simulink model "OFDM_Tx_HW"  (R2020a)
settings: Solver=FixedStepDiscrete  StartTime=0.0  StopTime=inf  RelTol=1e-3
InitFcn:
  | % Set parameters
  | fs = 20e6;
  | fclk = 240e6;
  | ssr = 2;
  | fdc = fclk*ssr*8;
  | 
  | % Load libraries
  | addpath('./lib');
  | 
  | % Create filters
  | run ./filter_design_20mhz;
  | 
  | % Load all required variables
  | load('variables/read_addr_data');
  | load('variables/read_addr_cp');
  | load('variables/read_addr_pream');
  | load('variables/read_addr_rx');
  | load('variables/pilot');
  | load('variables/sc_index');
  | load('variables/LTSfreq');
  | load('variables/STSfreq');
  | load('variables/LTSread');
  | load('variables/STSread');
  | 
  | run ./scripts/rfgen;
values from neighbouring files (symbols this model uses):
  decimation_unique = dsp.SampleRateConverter('InputSampleRate', fdc/64,     'OutputSampleRate', fs,     'Bandwidth', fs*0.9,     'OutputRateTolerance', 0,     'StopbandAttenuation', 100)    [filter_design_20mhz.m]
  interpolation_single = dsp.SampleRateConverter('InputSampleRate', fs,     'OutputSampleRate', fclk,     'Bandwidth', fs*0.9,     'OutputRateTolerance', 0,     'StopbandAttenuation', 100)    [filter_design_20mhz.m]
  interpolation_ssr = dsp.SampleRateConverter('InputSampleRate', fclk,     'OutputSampleRate', fclk*ssr,     'Bandwidth', fs*0.9,     'OutputRateTolerance', 0,     'StopbandAttenuation', 100)    [filter_design_20mhz.m]
undefined symbols (not defined in the file or in its folder): designMultirateFIR, LTSfreq, LTSread, pilot, read_addr_cp, read_addr_data, read_addr_pream, read_addr_rx, sc_index, STSfreq, STSread
libraries: hdlsllib x87, simulink x55, xbsIndex_r4 x48, dspmlti4 x23, xrbsSSR_Library x8, dspsigops x6, dspswit3 x4, dsphdlmathfun x3, dspsigattribs x2, dsphdlxfrm x2, dsphdlsigops x1, lib_rfsignalgenerator x1
(part 6 of 6)

== system OFDM_Tx_HW/OFDMTx/CPAdd/LTFExtend/LTFValidGen ==
  In1 : Inport
  AND : Logic  IconShape=distinctive  AllPortsSameDT=off  OutDataTypeStr=boolean
  AND1 : Logic  IconShape=distinctive  AllPortsSameDT=off  OutDataTypeStr=boolean
  Compare To Constant : simulink/Logic and Bit Operations/Compare To Constant  relop=>=  const=160  OutDataTypeStr=boolean
  Compare To Constant1 : simulink/Logic and Bit Operations/Compare To Constant  relop=<=  const=319  OutDataTypeStr=boolean
  HDL Counter : hdlsllib/Sources/HDL Counter  CountType=Count limited  CountInit=0  CountStep=1  CountMax=319  CountFromType=Initial value  CountFrom=0  CountResetPort=on  CountLoadPort=off  CountEnbPort=on  CountDirPort=off  CountDataType=Unsigned  CountWordLen=9  CountFracLen=0  CountSampTime=1
  NOT : Logic  Operator=NOT  IconShape=distinctive  AllPortsSameDT=off  OutDataTypeStr=boolean
  Out1 : Outport  VectorParamsAs1DForOutWhenUnconnected=off
  wires:
  Compare To Constant/1 -> AND/1
  In1/1 -> NOT/1, AND1/2, HDL Counter/2
  HDL Counter/1 -> Compare To Constant1/1, Compare To Constant/1
  Compare To Constant1/1 -> AND/2
  AND1/1 -> Out1/1
  AND/1 -> AND1/1
  NOT/1 -> HDL Counter/1

== system OFDM_Tx_HW/OFDMTx/CPAdd/LTFExtend/READ_CTRL ==
  In1 : Inport
  In2 : Inport  Port=2
  Constant : Constant  Value=0  OutDataTypeStr=fixdt(0,8,0)  SampleTime=1/fs
  Switch : Switch  Criteria=u2 ~= 0
  Out1 : Outport  VectorParamsAs1DForOutWhenUnconnected=off
  wires:
  Switch/1 -> Out1/1
  In1/1 -> Switch/1
  In2/1 -> Switch/2
  Constant/1 -> Switch/3

== system OFDM_Tx_HW/OFDMTx/CPAdd/STFExtend/READ_CTRL ==
  In1 : Inport
  In2 : Inport  Port=2
  Constant : Constant  Value=0  OutDataTypeStr=fixdt(0,8,0)  SampleTime=1/fs
  Switch : Switch  Criteria=u2 ~= 0
  Out1 : Outport  VectorParamsAs1DForOutWhenUnconnected=off
  wires:
  Constant/1 -> Switch/3
  In2/1 -> Switch/2
  In1/1 -> Switch/1
  Switch/1 -> Out1/1

== system OFDM_Tx_HW/OFDMTx/CPAdd/STFExtend/STFValidGen ==
  In1 : Inport
  AND : Logic  IconShape=distinctive  AllPortsSameDT=off  OutDataTypeStr=boolean
  AND1 : Logic  IconShape=distinctive  AllPortsSameDT=off  OutDataTypeStr=boolean
  Compare To Constant : simulink/Logic and Bit Operations/Compare To Constant  relop=>=  const=0  OutDataTypeStr=boolean
  Compare To Constant1 : simulink/Logic and Bit Operations/Compare To Constant  relop=<=  const=159  OutDataTypeStr=boolean
  HDL Counter : hdlsllib/Sources/HDL Counter  CountType=Count limited  CountInit=0  CountStep=1  CountMax=319  CountFromType=Initial value  CountFrom=0  CountResetPort=on  CountLoadPort=off  CountEnbPort=on  CountDirPort=off  CountDataType=Unsigned  CountWordLen=9  CountFracLen=0  CountSampTime=1
  NOT : Logic  Operator=NOT  IconShape=distinctive  AllPortsSameDT=off  OutDataTypeStr=boolean
  Out1 : Outport  VectorParamsAs1DForOutWhenUnconnected=off
  wires:
  Compare To Constant/1 -> AND/1
  In1/1 -> NOT/1, AND1/2, HDL Counter/2
  HDL Counter/1 -> Compare To Constant1/1, Compare To Constant/1
  Compare To Constant1/1 -> AND/2
  AND1/1 -> Out1/1
  AND/1 -> AND1/1
  NOT/1 -> HDL Counter/1

== system OFDM_Tx_HW/OFDMTx/ControlSignalGenerator/PreamValidGen/RisingEdge ==
  In1 : Inport
  Delay : Delay  DelayLength=1
  Relational Operator : RelationalOperator  Operator=>  OutDataTypeStr=boolean  RndMeth=Nearest
  Out1 : Outport
  wires:
  Relational Operator/1 -> Out1/1
  Delay/1 -> Relational Operator/2
  In1/1 -> Delay/1, Relational Operator/1

== system OFDM_Tx_HW/OFDMTx/DataGenerator/PilotGen/ToComplex1 ==
  In1 : Inport
  Constant1 : Constant  Value=0  OutDataTypeStr=fixdt(1,16,14)  SampleTime=1/fs
  Real-Imag to Complex : RealImagToComplex
  PilotOut : Outport  VectorParamsAs1DForOutWhenUnconnected=off
  wires:
  Constant1/1 -> Real-Imag to Complex/2
  In1/1 -> Real-Imag to Complex/1
  Real-Imag to Complex/1 -> PilotOut/1

== system OFDM_Tx_HW/OFDMTx/IFFT/IFFTValid/dataIFFTValid ==
  dataValidIn : Inport
  Compare To Constant : simulink/Logic and Bit Operations/Compare To Constant  relop=>=  const=17  OutDataTypeStr=boolean
  Logical Operator : Logic  Operator=NOT  IconShape=distinctive  AllPortsSameDT=off  OutDataTypeStr=boolean
  SAMPLE_COUNTER : hdlsllib/Sources/HDL Counter  CountType=Count limited  CountInit=1  CountStep=1  CountMax=80  CountFromType=Initial value  CountFrom=1  CountResetPort=on  CountLoadPort=off  CountEnbPort=on  CountDirPort=off  CountDataType=Unsigned  CountWordLen=7  CountFracLen=0  CountSampTime=1
  dataIFFTValidOut : Outport  VectorParamsAs1DForOutWhenUnconnected=off
  wires:
  dataValidIn/1 -> SAMPLE_COUNTER/2, Logical Operator/1
  Compare To Constant/1 -> dataIFFTValidOut/1
  Logical Operator/1 -> SAMPLE_COUNTER/1
  SAMPLE_COUNTER/1 -> Compare To Constant/1

== system OFDM_Tx_HW/OFDMTx/IFFT/IFFTValid/preambIFFTValid ==
  preambValid : Inport
  AND{,1..3} (4 alike) : Logic  IconShape=distinctive  AllPortsSameDT=off  OutDataTypeStr=boolean
  Compare To Constant1 : simulink/Logic and Bit Operations/Compare To Constant  relop=>=  const=96  OutDataTypeStr=boolean
  Compare To Constant2 : simulink/Logic and Bit Operations/Compare To Constant  relop=<=  const=159  OutDataTypeStr=boolean
  Compare To Constant3 : simulink/Logic and Bit Operations/Compare To Constant  relop=>=  const=256  OutDataTypeStr=boolean
  Compare To Constant4 : simulink/Logic and Bit Operations/Compare To Constant  relop=<=  const=319  OutDataTypeStr=boolean
  HDL Counter1 : hdlsllib/Sources/HDL Counter  CountType=Count limited  CountInit=0  CountStep=1  CountMax=319  CountFromType=Initial value  CountFrom=0  CountResetPort=on  CountLoadPort=off  CountEnbPort=on  CountDirPort=off  CountDataType=Unsigned  CountWordLen=9  CountFracLen=0  CountSampTime=1
  NOT : Logic  Operator=NOT  IconShape=distinctive  AllPortsSameDT=off  OutDataTypeStr=boolean
  OR : Logic  Operator=OR  IconShape=distinctive  AllPortsSameDT=off  OutDataTypeStr=boolean
  preambIFFTValidOut : Outport  VectorParamsAs1DForOutWhenUnconnected=off
  wires:
  AND/1 -> AND1/1
  AND2/1 -> AND3/1
  HDL Counter1/1 -> Compare To Constant4/1, Compare To Constant3/1, Compare To Constant2/1, Compare To Constant1/1
  OR/1 -> preambIFFTValidOut/1
  preambValid/1 -> HDL Counter1/2, AND3/2, AND1/2, NOT/1
  Compare To Constant1/1 -> AND/1
  Compare To Constant4/1 -> AND2/2
  AND1/1 -> OR/1
  AND3/1 -> OR/2
  Compare To Constant2/1 -> AND/2
  NOT/1 -> HDL Counter1/1
  Compare To Constant3/1 -> AND2/1

== system OFDM_Tx_HW/OFDMTx/SCMapper/DataMapper/READ_CTRL2 ==
  In1 : Inport
  In2 : Inport  Port=2
  Constant : Constant  Value=0  OutDataTypeStr=fixdt(0,8,0)  SampleTime=1/fs
  Switch : Switch  Criteria=u2 ~= 0
  Out1 : Outport  VectorParamsAs1DForOutWhenUnconnected=off
  wires:
  Switch/1 -> Out1/1
  In1/1 -> Switch/1
  In2/1 -> Switch/2
  Constant/1 -> Switch/3

== system OFDM_Tx_HW/OFDMTx/SCMapper/PremableMapper/READ_CTRL ==
  In1 : Inport
  In2 : Inport  Port=2
  Constant : Constant  Value=0  OutDataTypeStr=fixdt(0,8,0)  SampleTime=1/fs
  Switch : Switch  Criteria=u2 ~= 0
  Out1 : Outport  VectorParamsAs1DForOutWhenUnconnected=off
  wires:
  Switch/1 -> Out1/1
  In1/1 -> Switch/1
  In2/1 -> Switch/2
  Constant/1 -> Switch/3

== system OFDM_Tx_HW/decimate/Unique Decimation/Unique Decimation/FIR Decimator Unique ==
  Re Data In : Inport
  Im Data In : Inport  Port=2
  Convert7 : xbsIndex_r4/Convert  gui_display_data_type=Fixed-point  arith_type="Signed  (2's comp)"  n_bits=16  bin_pt=14  float_type=Single  exp_bits=8  fraction_bits=24  quantization="Round  (unbiased: +/- Inf)"  overflow=Saturate  en=off  latency=0  pipeline=off  dbl_ovrd=off  block_type=convert
  Convert8 : xbsIndex_r4/Convert  gui_display_data_type=Fixed-point  arith_type="Signed  (2's comp)"  n_bits=16  bin_pt=14  float_type=Single  exp_bits=8  fraction_bits=24  quantization="Round  (unbiased: +/- Inf)"  overflow=Saturate  en=off  latency=0  pipeline=off  dbl_ovrd=off  block_type=convert
  FIR Stage Unique : xbsIndex_r4/FIR Compiler 7.2   coefficientvector=decimation_unique.getFilters.Stage1.Numerator  coefficient_sets=1  coefficient_reload=off  filter_type=Decimation  rate_change_type=Integer  interpolation_rate=1  decimation_rate=decimation_unique.getFilters.Stage1.DecimationFactor  zero_pack_factor=1  channel_sequence=Basic  number_channels=1  pattern_list='P4-0,P4-1,P4-2,P4-3,P4-4'  number_paths=2  ratespecification=Maximum_Possible  sampleperiod=3  hardwareoversamplingrate=1  coefficient_sign=Signed  quantization=Quantize_Only  coefficient_width=16  bestprecision=on  coefficient_fractional_bits=16  coefficient_structure=Inferred  output_rounding_mode=Full_Precision  output_width=34  filter_architecture=Systolic_Multiply_Accumulate  optimization_goal=Area  optimization_list='None'  data_buffer_type=Automatic  coefficient_buffer_type=Automatic  input_buffer_type=Automatic  output_buffer_type=Automatic  preference_for_other_storage=Automatic  multi_column_support=Automatic  columnconfig='33'  inter_column_pipe_length=4  data_has_tlast=Not_Required  m_data_has_tready=off  s_data_has_fifo=off  s_data_has_tuser=Not_Required  m_data_has_tuser=Not_Required  s_config_sync_mode=On_Vector  s_config_method=Single  num_reload_slots=1  has_aclken=off  has_aresetn=off  infoeditControl=ARESETn must be asserted for a minimum of 2 cycles  reset_data_vector=on  trim_axipin_name=on  simulation_type=hybrid_sim  simulation_model=sysgen:xfirv7_2_cmodel  data_path_portlist={ 's_axis_data_tdata', 'm_axis_data_tdata' }  passband_min=0.0  passband_max=0.5  stopband_min=0.5  stopband_max=1.0  filter_selection=1  gui_behaviour='Sysgen_GUI'  data_sign=Signed  data_width=16  data_fractional_bits=0  data_tuser_width=1  wrapper_available=true  ip_wrap_arbitrary_binary_point=true  ip_name=FIR Compiler  ip_version=7.2  dsptool_ready=true  ipcore_usecache=true  ipcore_useipmodelcache=true  port_translation_map={ 'aclken' => 'en', 'aresetn' => 'rst' }  run_core_at_system_period=true  ipcore_xco_need_fpga_part=true  block_type=fir_compiler_v7_2
      settings: infoedit=Maximum Possible : Maximizes oversampling rate. Abstracted input handshake (no s_data_tvalid) and automatic rate propagation.<br>Hardware Oversampling Rate : Specifies oversampling rate relative to the input sample period. Abstracted input handshake (no s_data_tvalid) and automatic rate propagation.<br>Input/Output Sample Period : Specifies absolute oversampling rate. No input handshake abstraction (exposes s_data_tvalid) and no rate propagation.
  Terminator5 : Terminator
  Terminator6 : Terminator
  Re Data Out : Outport
  Im Data Out : Outport  Port=2
  wires:
  FIR Stage Unique/1 -> Terminator6/1
  FIR Stage Unique/2 -> Terminator5/1
  FIR Stage Unique/3 -> Convert7/1
  FIR Stage Unique/4 -> Convert8/1
  Im Data In/1 -> FIR Stage Unique/2
  Convert8/1 -> Im Data Out/1
  Re Data In/1 -> FIR Stage Unique/1
  Convert7/1 -> Re Data Out/1

== system OFDM_Tx_HW/Channel/RF-ADC/NCO and Mixer/RF-ADC Coarse Mixer/Negate ==
  Data In : Inport
  Complex to Real-Imag2 : ComplexToRealImag
  Real-Imag to Complex1 : RealImagToComplex
  Unary Minus : UnaryMinus
  Data Out : Outport  VectorParamsAs1DForOutWhenUnconnected=off
  wires:
  Complex to Real-Imag2/2 -> Unary Minus/1
  Unary Minus/1 -> Real-Imag to Complex1/2
  Data In/1 -> Complex to Real-Imag2/1
  Real-Imag to Complex1/1 -> Data Out/1
  Complex to Real-Imag2/1 -> Real-Imag to Complex1/1

== system OFDM_Tx_HW/Channel/RF-ADC/NCO and Mixer/RF-ADC Coarse Mixer/fs_2 ==
  Data In : Inport
  Counter : dspswit3/Counter  Direction=Up  CountEvent=Free running  CounterSize=User defined  MaxCount=1  InitialCount=0  Output=Count  HitValue=32  ResetInput=off  SamplesPerFrame=ssr  Ts=1/(fs)  CntDtype=uint8  HitDtype=Logical
  Multiport Switch2 : MultiPortSwitch  DataPortOrder=Zero-based contiguous  Inputs=2  zeroidx=on
  Real-Imag to Complex : RealImagToComplex
  Real-Imag to Complex1 : RealImagToComplex
  Unary Minus1 : UnaryMinus
  Data Out : Outport  VectorParamsAs1DForOutWhenUnconnected=off
  wires:
  Data In/1 -> Real-Imag to Complex1/1, Real-Imag to Complex1/2, Unary Minus1/1
  Real-Imag to Complex1/1 -> Multiport Switch2/2
  Real-Imag to Complex/1 -> Multiport Switch2/3
  Multiport Switch2/1 -> Data Out/1
  Counter/1 -> Multiport Switch2/1
  Unary Minus1/1 -> Real-Imag to Complex/2, Real-Imag to Complex/1

== system OFDM_Tx_HW/Channel/RF-ADC/NCO and Mixer/RF-ADC Coarse Mixer/fs_4 ==
  note: Real:	1, 0, -1, 0
      | Imag:	0, 1, 0, -1
  Data In : Inport
  Counter : dspswit3/Counter  Direction=Up  CountEvent=Free running  CounterSize=User defined  MaxCount=3  InitialCount=0  Output=Count  HitValue=32  ResetInput=off  SamplesPerFrame=ssr  Ts=1/(fs)  CntDtype=uint8  HitDtype=Logical
  Multiport Switch2 : MultiPortSwitch  DataPortOrder=Zero-based contiguous  Inputs=4  zeroidx=on
  Real-Imag to Complex{1..4} (4 alike) : RealImagToComplex
  Unary Minus : UnaryMinus
  Unary Minus1 : UnaryMinus
  Unary Minus2 : UnaryMinus
  Data Out : Outport  VectorParamsAs1DForOutWhenUnconnected=off
  wires:
  Unary Minus/1 -> Real-Imag to Complex3/1
  Unary Minus2/1 -> Real-Imag to Complex2/2
  Real-Imag to Complex4/1 -> Multiport Switch2/2
  Unary Minus1/1 -> Real-Imag to Complex1/2, Real-Imag to Complex1/1
  Real-Imag to Complex1/1 -> Multiport Switch2/4
  Counter/1 -> Multiport Switch2/1
  Real-Imag to Complex2/1 -> Multiport Switch2/3
  Data In/1 -> Real-Imag to Complex4/1, Unary Minus2/1, Unary Minus1/1, Unary Minus/1, Real-Imag to Complex3/2, Real-Imag to Complex2/1, Real-Imag to Complex4/2
  Real-Imag to Complex3/1 -> Multiport Switch2/5
  Multiport Switch2/1 -> Data Out/1

== system OFDM_Tx_HW/Channel/RF-DAC/NCO and Mixer/RF-DAC Coarse Mixer/Negate ==
  Data In : Inport
  Complex to Real-Imag2 : ComplexToRealImag
  Real-Imag to Complex1 : RealImagToComplex
  Unary Minus : UnaryMinus
  Data Out : Outport  VectorParamsAs1DForOutWhenUnconnected=off
  wires:
  Complex to Real-Imag2/1 -> Real-Imag to Complex1/1
  Real-Imag to Complex1/1 -> Data Out/1
  Data In/1 -> Complex to Real-Imag2/1
  Unary Minus/1 -> Real-Imag to Complex1/2
  Complex to Real-Imag2/2 -> Unary Minus/1

== system OFDM_Tx_HW/Channel/RF-DAC/NCO and Mixer/RF-DAC Coarse Mixer/fs_2 ==
  Data In : Inport
  Counter : dspswit3/Counter  Direction=Up  CountEvent=Free running  CounterSize=User defined  MaxCount=1  InitialCount=0  Output=Count  HitValue=32  ResetInput=off  SamplesPerFrame=ssr  Ts=1/(fs)  CntDtype=uint8  HitDtype=Logical
  Multiport Switch2 : MultiPortSwitch  DataPortOrder=Zero-based contiguous  Inputs=2  zeroidx=on
  Unary Minus : UnaryMinus
  Data Out : Outport  VectorParamsAs1DForOutWhenUnconnected=off
  wires:
  Multiport Switch2/1 -> Data Out/1
  Counter/1 -> Multiport Switch2/1
  Unary Minus/1 -> Multiport Switch2/3
  Data In/1 -> Multiport Switch2/2, Unary Minus/1

== system OFDM_Tx_HW/Channel/RF-DAC/NCO and Mixer/RF-DAC Coarse Mixer/fs_4 ==
  note: Real:	1, 0, -1, 0
      | Imag:	0, 1, 0, -1
  Data In : Inport
  Complex to Real-Imag : ComplexToRealImag
  Complex to Real-Imag1 : ComplexToRealImag
  Counter : dspswit3/Counter  Direction=Up  CountEvent=Free running  CounterSize=User defined  MaxCount=3  InitialCount=0  Output=Count  HitValue=32  ResetInput=off  SamplesPerFrame=ssr  Ts=1/(fs)  CntDtype=uint8  HitDtype=Logical
  Multiport Switch2 : MultiPortSwitch  DataPortOrder=Zero-based contiguous  Inputs=4  zeroidx=on
  Real-Imag to Complex2 : RealImagToComplex
  Real-Imag to Complex3 : RealImagToComplex
  Unary Minus : UnaryMinus
  Unary Minus1 : UnaryMinus
  Unary Minus2 : UnaryMinus
  Data Out : Outport  VectorParamsAs1DForOutWhenUnconnected=off
  wires:
  Unary Minus2/1 -> Real-Imag to Complex2/1
  Complex to Real-Imag/2 -> Unary Minus2/1
  Unary Minus/1 -> Real-Imag to Complex3/2
  Complex to Real-Imag1/1 -> Unary Minus/1
  Complex to Real-Imag1/2 -> Real-Imag to Complex3/1
  Multiport Switch2/1 -> Data Out/1
  Real-Imag to Complex3/1 -> Multiport Switch2/5
  Data In/1 -> Multiport Switch2/2, Complex to Real-Imag/1, Complex to Real-Imag1/1, Unary Minus1/1
  Unary Minus1/1 -> Multiport Switch2/4
  Complex to Real-Imag/1 -> Real-Imag to Complex2/2
  Real-Imag to Complex2/1 -> Multiport Switch2/3
  Counter/1 -> Multiport Switch2/1

== system OFDM_Tx_HW/OFDMRx/PhaseTracking_1/PilotCtrlGen/pilotGen/ToComplex1 ==
  In1 : Inport
  Constant1 : Constant  Value=0  OutDataTypeStr=fixdt(1,2,0)  SampleTime=1/fs
  Real-Imag to Complex : RealImagToComplex
  Out1 : Outport  VectorParamsAs1DForOutWhenUnconnected=off
  wires:
  Constant1/1 -> Real-Imag to Complex/2
  In1/1 -> Real-Imag to Complex/1
  Real-Imag to Complex/1 -> Out1/1

== system OFDM_Tx_HW/OFDMRx/PhaseTracking_2/PilotCtrlGen/pilotGen/ToComplex1 ==
  In1 : Inport
  Constant1 : Constant  Value=0  OutDataTypeStr=fixdt(1,2,0)  SampleTime=1/fs
  Real-Imag to Complex : RealImagToComplex
  Out1 : Outport  VectorParamsAs1DForOutWhenUnconnected=off
  wires:
  Constant1/1 -> Real-Imag to Complex/2
  In1/1 -> Real-Imag to Complex/1
  Real-Imag to Complex/1 -> Out1/1

== system OFDM_Tx_HW/OFDMRx/Synchronisation/ControlSigGen/PreambleValidGen/RisingEdge ==
  ValidIn : Inport
  Delay : Delay  DelayLength=1
  Relational Operator : RelationalOperator  Operator=>  OutDataTypeStr=boolean  RndMeth=Nearest
  Out1 : Outport
  wires:
  ValidIn/1 -> Relational Operator/1, Delay/1
  Delay/1 -> Relational Operator/2
  Relational Operator/1 -> Out1/1

== matlab function OFDM_Tx_HW/OFDMRx/PhaseTracking_1/CordicRotate/QCORR/QUAD_MAP1 ==
  data: xin input; xout output; yout output; yin input; ctrl input
function [xout,yout] = fcn(xin,yin,ctrl)
% Process to perform final rotation 
% by pi/2 if the original angle was 
% in 3rd or 4th quadrants    
if ctrl == 0
    % 1st or 2nd quadrants 
    xout = fi(xin,1,21,15);  
    yout = fi(yin,1,21,15);  
elseif ctrl == 1
    % 3rd quadrant (rotate pi/2 clockwise)
    xout = fi(yin,1,21,15); 
    yout = fi(-xin,1,21,15); 
elseif ctrl == 2
    % 4th quadrant (rotate pi/2 anti-clockwise) 
    xout = fi(-yin,1,21,15); 
    yout = fi(xin,1,21,15); 
else 
    % others clause
    xout = fi(xin,1,21,15); 
    yout = fi(yin,1,21,15); 
end

== matlab function OFDM_Tx_HW/OFDMTx/DataGenerator/Data Multiplexer ==
  data: symbols input; dataready input; data output; pilots input; pval input; sts input; stsval input; lts input; ltsval input
function data  = dataMux(symbols,dataready,pilots,pval,sts,stsval,lts,ltsval)
% Data multiplexer 
if (pval == true)
    data = pilots; 
elseif (stsval == true)
    data = sts; 
elseif (ltsval == true)
    data = lts; 
elseif (dataready == true) 
    data = symbols;
else 
    data = fi(complex(0),1,16,14);
end

== matlab function OFDM_Tx_HW/OFDMRx/PhaseTracking_1/CordicRotate/QUAD_MAP/QUAD_DETERM1 ==
  data: ang_in input; ang_out output; QUAD output
function [ang_out,QUAD] = fcn(ang_in)
% Process to determine quadrant and 
% shift into region -pi/2 to pi/2 if 
% not already there 
v = fi(pi,1,23,20);
x = fi(-pi,1,23,20); 
y = fi(-pi/2,1,23,20); 
z = fi(pi/2,1,23,20);

% Determine quadrant 
if ((ang_in >= y) && (ang_in <= z))
    QUAD = fi(0,0,2,0); % Quads 1 or 2
elseif ((ang_in < y) && (ang_in >= x))
    QUAD = fi(1,0,2,0); % Quad 3
elseif ((ang_in > z) && (ang_in <= v))
    QUAD = fi(2,0,2,0); % Quad 4
else 
    % others clause
    QUAD = fi(0,0,2,0);
end 

% Determine whether we need to add or subtract pi/2 
% based on quadrant location
switch(QUAD) 
    
    case 0 
        % Angle stays the same 
        ang_out = fi(ang_in, 1, 23, 20); 
    case 1
        % pi/2 is added to angle (anti-clockwise)
        ang_out = fi(ang_in + z, 1, 23, 20); 
    case 2
        % pi/2 is subtracted from angle (clockwise)
        ang_out = fi(ang_in - z, 1, 23, 20); 
    otherwise
        % others clause make output angle 
        % equal to input angle  
        ang_out = fi(ang_in, 1, 23, 20); 
end

== matlab function OFDM_Tx_HW/OFDMTx/CPAdd/Mux2 ==
  data: sts input; stsval input; lts input; ltsval input; dataOut output; data input; dataval input
function dataOut = mux(sts,stsval,lts,ltsval,data,dataval)

if (stsval == true)
    dataOut = sts; 
elseif (ltsval == true)
    dataOut = lts; 
elseif (dataval == true) 
    dataOut = data; 
else 
    dataOut = fi(complex(0),1,16,14);
end

== matlab function OFDM_Tx_HW/OFDMTx/SCMapper/Mux2 ==
  data: preamb input; preambVal input; dataOut output; data input; dataVal input
function dataOut = mux(preamb,preambVal,data,dataVal)

if (preambVal == true)
    dataOut = preamb; 
elseif (dataVal == true)
    dataOut = data; 
else 
    dataOut = fi(complex(0),1,16,14);
end

== matlab function OFDM_Tx_HW/OFDMRx/PhaseTracking_2/CordicRotate/QCORR/QUAD_MAP1 ==
  data: xin input; xout output; yout output; yin input; ctrl input
function [xout,yout] = fcn(xin,yin,ctrl)
% Process to perform final rotation 
% by pi/2 if the original angle was 
% in 3rd or 4th quadrants    
if ctrl == 0
    % 1st or 2nd quadrants 
    xout = fi(xin,1,21,15);  
    yout = fi(yin,1,21,15);  
elseif ctrl == 1
    % 3rd quadrant (rotate pi/2 clockwise)
    xout = fi(yin,1,21,15); 
    yout = fi(-xin,1,21,15); 
elseif ctrl == 2
    % 4th quadrant (rotate pi/2 anti-clockwise) 
    xout = fi(-yin,1,21,15); 
    yout = fi(xin,1,21,15); 
else 
    % others clause
    xout = fi(xin,1,21,15); 
    yout = fi(yin,1,21,15); 
end

== matlab function OFDM_Tx_HW/OFDMRx/PhaseTracking_2/CordicRotate/QUAD_MAP/QUAD_DETERM1 ==
  data: ang_in input; ang_out output; QUAD output
function [ang_out,QUAD] = fcn(ang_in)
% Process to determine quadrant and 
% shift into region -pi/2 to pi/2 if 
% not already there 
v = fi(pi,1,23,20);
x = fi(-pi,1,23,20); 
y = fi(-pi/2,1,23,20); 
z = fi(pi/2,1,23,20);

% Determine quadrant 
if ((ang_in >= y) && (ang_in <= z))
    QUAD = fi(0,0,2,0); % Quads 1 or 2
elseif ((ang_in < y) && (ang_in >= x))
    QUAD = fi(1,0,2,0); % Quad 3
elseif ((ang_in > z) && (ang_in <= v))
    QUAD = fi(2,0,2,0); % Quad 4
else 
    % others clause
    QUAD = fi(0,0,2,0);
end 

% Determine whether we need to add or subtract pi/2 
% based on quadrant location
switch(QUAD) 
    
    case 0 
        % Angle stays the same 
        ang_out = fi(ang_in, 1, 23, 20); 
    case 1
        % pi/2 is added to angle (anti-clockwise)
        ang_out = fi(ang_in + z, 1, 23, 20); 
    case 2
        % pi/2 is subtracted from angle (clockwise)
        ang_out = fi(ang_in - z, 1, 23, 20); 
    otherwise
        % others clause make output angle 
        % equal to input angle  
        ang_out = fi(ang_in, 1, 23, 20); 
end
